simulink model "TCM8AMPM_4QAM"  (Simulink 10.2)
settings: Solver=VariableStepDiscrete  StartTime=0.0  StopTime=1e5  RelTol=1e-3  EnableMultiTasking=on
model workspace (MAT data in the model file):
  A = 1
  BER_exit = 0.0020497950205
  BER_th = 0.001
  K = 4
  M = 8
  N = 50
  P_TCM = 10
  P_UNCODED = 2
  T = 1
  ber_TCM = [0.36658979244 0.35791637421 0.332748420736 0.291837962499 0.223052241051 0.119372305224 0.0331896119523 0.00376015241151 0.000300812192921 0.000100270730974]
  ber_UNCODED = [0.163933606639 0.133536646335 0.104839516048 0.0776922307769 0.0546445355464 0.035696430357 0.0220477952205 0.012398760124 0.00599940005999 0.0020497950205]
  ber_tcm_bit_coded = [0.423343026171 0.416825428657 0.395217086133 0.359671112002 0.293291888098 0.173568635315 0.0536448410709 0.00681840970621 0 0]
  ber_tcm_bit_uncoded = [0.104791258055 0.0724912090885 0.0548450565667 0.0454348766768 0.0279695521331 0.0128376571276 0.00521455730581 0.00212593642438 0.000601624385842 0.000200541461947]
  coded_bit = 2
  coded_bit_conv = [2 3]
  codegen = [1  0  0; 0  133  171]
  codegen_2 = [133 171]
  constlen = [1 7]
  constlen_2 = 7
  generator_c1 = 133
  generator_c2 = 171
  h = 22
  hh = 0
  hws = Simulink.ModelWorkspace
  i = 11
  k = 2
  label_coded = 'TCM8AMPM'
  label_uncoded = '4QAM'
  list : struct (value not decoded)
  m = 3
  mapping_tcm = [-1+3i 3-1i 3+3i -1-1i -3+1i 1-3i 1+1i -3-3i]
  mdl_name = 'TCM8AMPM_4QAM'
  mm = 0
  n = 10000
  num_states = 64
  register_length = 7
  seed = 208004
  snr = 10
  snr_start = 0
  snr_step = 1
  snr_vec = [0 1 2 3 4 5 6 7 8 9 10]
  ss = 0.49
  startTime = [2021 6 12 8 24 9.036]
  stepTime = [2021 6 12 8 25 8.076]
  step_dur = 0.49
  tb = 28
  tout = [9001 9002 9003 9004 9005 9006 9007 9008 9009 9010 9011 9012 ... (1000 elements, 1000x1)]
  trellis.numInputSymbols = 4
  trellis.numOutputSymbols = 8
  trellis.numStates = 64
  trellis.nextStates = [0  32  0  32; 0  32  0  32; 1  33  1  33; 1  33  1  33; 2  34  2  34; 2  34  2  34; 3  35  3  35; 3  35  3  35; 4  36  4  36; 4  36  4  36; 5  37  5  37; 5  37  5  37; 6  38  6  38; 6  38  6  38; 7  39  7  39; 7  39  7  39; 8  40  8  40; 8  40  8  40; 9  41  9  41; 9  41  9  41; 10  42  10  42; 10  42  10  42; 11  43  11  43; 11  43  11  43; 12  44  12  44; 12  44  12  44; 13  45  13  45; 13  45  13  45; 14  46  14  46; 14  46  14  46; 15  47  15  47; 15  47  15  47; 16  48  16  48; 16  48  16  48; 17  49  17  49; 17  49  17  49; 18  50  18  50; 18  50  18  50; 19  51  19  51; 19  51  19  51; 20  52  20  52; 20  52  20  52; 21  53  21  53; 21  53  21  53; 22  54  22  54; 22  54  22  54; 23  55  23  55; 23  55  23  55; 24  56  24  56; 24  56  24  56; 25  57  25  57; 25  57  25  57; 26  58  26  58; 26  58  26  58; 27  59  27  59; 27  59  27  59; 28  60  28  60; 28  60  28  60; 29  61  29  61; 29  61  29  61; 30  62  30  62; 30  62  30  62; 31  63  31  63; 31  63  31  63]
  trellis.outputs = [0  3  4  7; 3  0  7  4; 2  1  6  5; 1  2  5  6; 0  3  4  7; 3  0  7  4; 2  1  6  5; 1  2  5  6; 3  0  7  4; 0  3  4  7; 1  2  5  6; 2  1  6  5; 3  0  7  4; 0  3  4  7; 1  2  5  6; 2  1  6  5; 3  0  7  4; 0  3  4  7; 1  2  5  6; 2  1  6  5; 3  0  7  4; 0  3  4  7; 1  2  5  6; 2  1  6  5; 0  3  4  7; 3  0  7  4; 2  1  6  5; 1  2  5  6; 0  3  4  7; 3  0  7  4; 2  1  6  5; 1  2  5  6; 1  2  5  6; 2  1  6  5; 3  0  7  4; 0  3  4  7; 1  2  5  6; 2  1  6  5; 3  0  7  4; 0  3  4  7; 2  1  6  5; 1  2  5  6; 0  3  4  7; 3  0  7  4; 2  1  6  5; 1  2  5  6; 0  3  4  7; 3  0  7  4; 2  1  6  5; 1  2  5  6; 0  3  4  7; 3  0  7  4; 2  1  6  5; 1  2  5  6; 0  3  4  7; 3  0  7  4; 1  2  5  6; 2  1  6  5; 3  0  7  4; 0  3  4  7; 1  2  5  6; 2  1  6  5; 3  0  7  4; 0  3  4  7]
  trellis_2.numInputSymbols = 2
  trellis_2.numOutputSymbols = 4
  trellis_2.numStates = 64
  trellis_2.nextStates = [0  32; 0  32; 1  33; 1  33; 2  34; 2  34; 3  35; 3  35; 4  36; 4  36; 5  37; 5  37; 6  38; 6  38; 7  39; 7  39; 8  40; 8  40; 9  41; 9  41; 10  42; 10  42; 11  43; 11  43; 12  44; 12  44; 13  45; 13  45; 14  46; 14  46; 15  47; 15  47; 16  48; 16  48; 17  49; 17  49; 18  50; 18  50; 19  51; 19  51; 20  52; 20  52; 21  53; 21  53; 22  54; 22  54; 23  55; 23  55; 24  56; 24  56; 25  57; 25  57; 26  58; 26  58; 27  59; 27  59; 28  60; 28  60; 29  61; 29  61; 30  62; 30  62; 31  63; 31  63]
  trellis_2.outputs = [0  3; 3  0; 2  1; 1  2; 0  3; 3  0; 2  1; 1  2; 3  0; 0  3; 1  2; 2  1; 3  0; 0  3; 1  2; 2  1; 3  0; 0  3; 1  2; 2  1; 3  0; 0  3; 1  2; 2  1; 0  3; 3  0; 2  1; 1  2; 0  3; 3  0; 2  1; 1  2; 1  2; 2  1; 3  0; 0  3; 1  2; 2  1; 3  0; 0  3; 2  1; 1  2; 0  3; 3  0; 2  1; 1  2; 0  3; 3  0; 2  1; 1  2; 0  3; 3  0; 2  1; 1  2; 0  3; 3  0; 1  2; 2  1; 3  0; 0  3; 1  2; 2  1; 3  0; 0  3]
  uncoded_bit = 1
undefined symbols (not defined in the file): Mnum
libraries: commsink2 x4, commutil2 x4, dspindex x4, commdigbbndam3 x3, commchan3 x2, commcnvcod2 x2, commdigbbndtcm2 x1, commrandsrc2 x1
settings Model: Creator=Diego  LastModifiedBy=diego
settings DataIOCC: LimitDataPoints=on
settings OptimizationCC: ExpressionDepthLimit=2147483647
settings DebuggingCC: SolverPrmCheckMsg=warning  StateNameClashWarn=warning
settings GRTTargetCC: CombineOutputUpdateFcns=on  GRTInterface=off

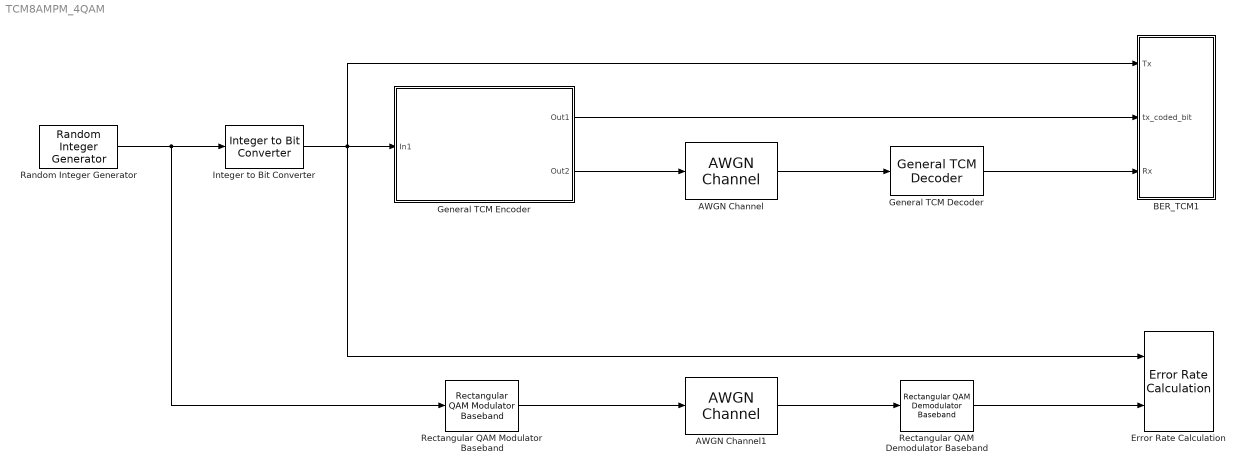
== system TCM8AMPM_4QAM ==
  AWGN Channel : commchan3/AWGN Channel  InputProcessing=Columns as channels (frame based)  seed=seed  noiseMode="Signal to noise ratio  (Es/No)"  EbNodB=Eb_No  EsNodB=snr  SNRdB=snr  bitsPerSym=k  Ps=P_TCM  Tsym=T  variance=1
  AWGN Channel1 : commchan3/AWGN Channel  InputProcessing=Columns as channels (frame based)  seed=seed  noiseMode="Signal to noise ratio  (Es/No)"  EbNodB=Eb_No  EsNodB=snr  SNRdB=snr  bitsPerSym=k  Ps=P_UNCODED  Tsym=T  variance=1
  BER_TCM1 : Subsystem
  Error Rate Calculation : commsink2/Error Rate Calculation  N=0  st_delay=0  cp_mode=Entire frame  subframe=[]  PMode=Workspace  WsName=ErrorVec_UNCODED  RsMode2=off  stop=off  numErr=100  maxBits=1e7
  General TCM Decoder : commdigbbndtcm2/General TCM Decoder  trellis=trellis  constpts=mapping_tcm  tbdepth=tb  opmode=Continuous  reset=off  outDtype=double
      settings: SourceProductBaseCode=CM
  General TCM Encoder : Subsystem  AncestorBlock=commdigbbndtcm2/General TCM Encoder  mask(General TCM Encoder){trellis=trellis, opMode=Continuous, constpts=mapping_tcm, outDtype=double}
      mask prompts: trellis "Trellis structure:"; opMode "Operation mode:"; constpts "Signal constellation:"; outDtype "Output data type"
      mask help:
      | Convolutionally encode binary data and perform signal mapping using the Signal constellation parameter, which expects complex constellation points in the set-partitioned order.
      |
      | The Trellis structure parameter must be a valid MATLAB trellis structure. To check if a structure is a valid trellis structure, use the istrellis function in MATLAB.
      mask init:
      | [constpts, Mnum, err, inPortLbl, rstPortLbl] = commblkgentcmenc(gcb, 'init', trellis, constpts);
      | if ~isempty(err.msg)
      | 	error(err.mmi,err.msg);
      | end
      mask Help: helpview(commbhelp)
      mask TypeOptions opMode: Continuous | Truncated (reset every frame) | Terminate trellis by appending bits | Reset on nonzero input via port
      mask TypeOptions outDtype: double | single
      mask Callback outDtype: commblkgentcmenc(gcb, 'cbDtype');
      mask Display:
      | disp('General\nTCM');
      | text(inPortLbl.x, inPortLbl.y, inPortLbl.str);
      | text(rstPortLbl.x, rstPortLbl.y, rstPortLbl.str);
  Integer to Bit Converter : commutil2/Integer to Bit Converter  nbits=2  signedInputValues=Unsigned  bitOrder=MSB first  outDtype=Inherit via internal rule
  Random Integer Generator : commrandsrc2/Random Integer Generator  mul=4  seed=10  Ts=1  frameBased=off  sampPerFrame=1000  orient=off  outDataType=double
      settings: SourceProductBaseCode=CM
  Rectangular QAM Demodulator Baseband : commdigbbndam3/Rectangular QAM Demodulator Baseband  M=4  OutType=Bit  DecType=Hard decision  VarSource=Dialog  Variance=1  Dec=Gray  Mapping=[0:15]  PowType=Min. distance between symbols  MinDist=2  AvgPow=1  PeakPow=1  Ph=0  outDtype1=Inherit via internal rule  outDtype2=Inherit via internal rule  derotateFactorWordLen=16  derotateFactorDataTypeStr=Inherit: Same word length as input  derotateFactorLastDataTypeStr=Inherit: Same word length as input  denormFactorWordLen=16  denormFactorDataTypeStr=Inherit: Same word length as input  denormFactorLastDataTypeStr=Inherit: Same word length as input  prodOutWordLen=32  prodOutOverflowMode=Wrap  prodOutRoundingMode=Floor  prodOutOvFlMode=off  prodOutOvFlModeLastStrValue=off  sumWordLen=32
  Rectangular QAM Modulator Baseband : commdigbbndam3/Rectangular QAM Modulator Baseband  M=4  InType=Integer  Enc=Gray  Mapping=[0:15]  PowType=Min. distance between symbols  MinDist=2  AvgPow=1  PeakPow=1  Ph=0  outDtype=double  outWordLen=16  outUDDataType=sfix(16)  outFracLenMode=Best precision  outFracLen=15  outDataTypeStr=double  outLastDataTypeStr=double
  wires:
  Integer to Bit Converter/1 -> Error Rate Calculation/1, General TCM Encoder/1(In1), BER_TCM1/1(Tx)
  Random Integer Generator/1 -> Rectangular QAM Modulator Baseband/1, Integer to Bit Converter/1
  AWGN Channel/1 -> General TCM Decoder/1
  General TCM Decoder/1 -> BER_TCM1/3(Rx)
  Rectangular QAM Modulator Baseband/1 -> AWGN Channel1/1
  AWGN Channel1/1 -> Rectangular QAM Demodulator Baseband/1
  Rectangular QAM Demodulator Baseband/1 -> Error Rate Calculation/2
  General TCM Encoder/2(Out2) -> AWGN Channel/1
  General TCM Encoder/1(Out1) -> BER_TCM1/2(tx_coded_bit)

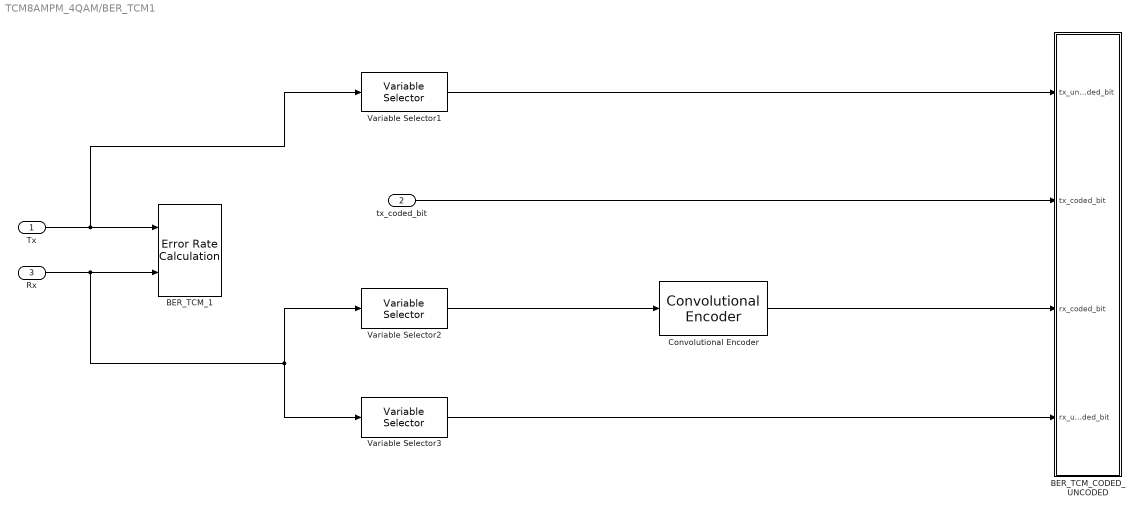
== system TCM8AMPM_4QAM/BER_TCM1 ==
  Tx : Inport
  tx_coded_bit : Inport  Port=2
  Rx : Inport  Port=3
  BER_TCM_1 : commsink2/Error Rate Calculation  N=tb*k  st_delay=0  cp_mode=Entire frame  subframe=[]  PMode=Workspace  WsName=ErrorVec_TCM_1  RsMode2=off  stop=off  numErr=100  maxBits=1e6
  BER_TCM_CODED_UNCODED : Subsystem
  Convolutional Encoder : commcnvcod2/Convolutional Encoder  trellis=trellis_2  opMode=Continuous  DelayedResetAction=off  hasIniStPort=off  hasFinStPort=off  usePuncVector=off  punctureVector=[1; 1; 0; 1; 0; 1]  reset=Unused parameter value
      settings: SourceProductBaseCode=CM
  Variable Selector1 : dspindex/Variable Selector  NumInputs=1  rowsOrCols=Rows  IdxMode=Fixed  Elements=uncoded_bit  ZerOneIdxMode=One-based  errmode=Clip Index  FillMode=on  FillValues=0
  Variable Selector2 : dspindex/Variable Selector  NumInputs=1  rowsOrCols=Rows  IdxMode=Fixed  Elements=coded_bit  ZerOneIdxMode=One-based  errmode=Clip Index  FillMode=on  FillValues=0
  Variable Selector3 : dspindex/Variable Selector  NumInputs=1  rowsOrCols=Rows  IdxMode=Fixed  Elements=uncoded_bit  ZerOneIdxMode=One-based  errmode=Clip Index  FillMode=on  FillValues=0
  wires:
  Tx/1 -> BER_TCM_1/1, Variable Selector1/1
  Rx/1 -> BER_TCM_1/2, Variable Selector2/1, Variable Selector3/1
  Variable Selector1/1 -> BER_TCM_CODED_UNCODED/1(tx_uncoded_bit)
  Variable Selector2/1 -> Convolutional Encoder/1
  Variable Selector3/1 -> BER_TCM_CODED_UNCODED/4(rx_uncoded_bit)
  tx_coded_bit/1 -> BER_TCM_CODED_UNCODED/2(tx_coded_bit)
  Convolutional Encoder/1 -> BER_TCM_CODED_UNCODED/3(rx_coded_bit)

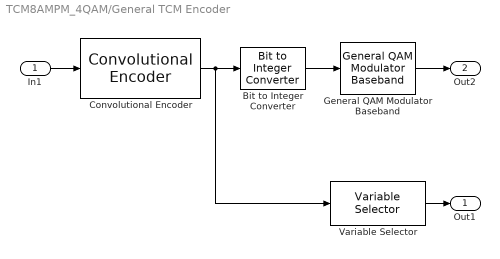
== system TCM8AMPM_4QAM/General TCM Encoder ==
  In1 : Inport
  Bit to Integer Converter : commutil2/Bit to Integer Converter  nbits=log2(Mnum)  bitOrder=MSB first  signedOutputValues=Unsigned  outDtype=uint32  outDtypeSigned=Inherit via internal rule
  Convolutional Encoder : commcnvcod2/Convolutional Encoder  trellis=trellis  opMode=Continuous  DelayedResetAction=off  hasIniStPort=off  hasFinStPort=off  usePuncVector=off  punctureVector=[1; 1; 0; 1; 0; 1]  reset=Unused parameter value
      settings: SourceProductBaseCode=CM
  General QAM Modulator Baseband : commdigbbndam3/General QAM Modulator Baseband  SigCon=constpts  outDtype=double  outWordLen=16  outUDDataType=sfix(16)  outFracLenMode=Best precision  outFracLen=15  outDataTypeStr=double  outLastDataTypeStr=double
      settings: SourceProductBaseCode=CM
  Variable Selector : dspindex/Variable Selector  NumInputs=1  rowsOrCols=Rows  IdxMode=Fixed  Elements=coded_bit_conv  ZerOneIdxMode=One-based  errmode=Clip Index  FillMode=on  FillValues=0
  Out1 : Outport
  Out2 : Outport  Port=2
  wires:
  Bit to Integer Converter/1 -> General QAM Modulator Baseband/1
  In1/1 -> Convolutional Encoder/1
  Convolutional Encoder/1 -> Bit to Integer Converter/1, Variable Selector/1
  General QAM Modulator Baseband/1 -> Out2/1
  Variable Selector/1 -> Out1/1

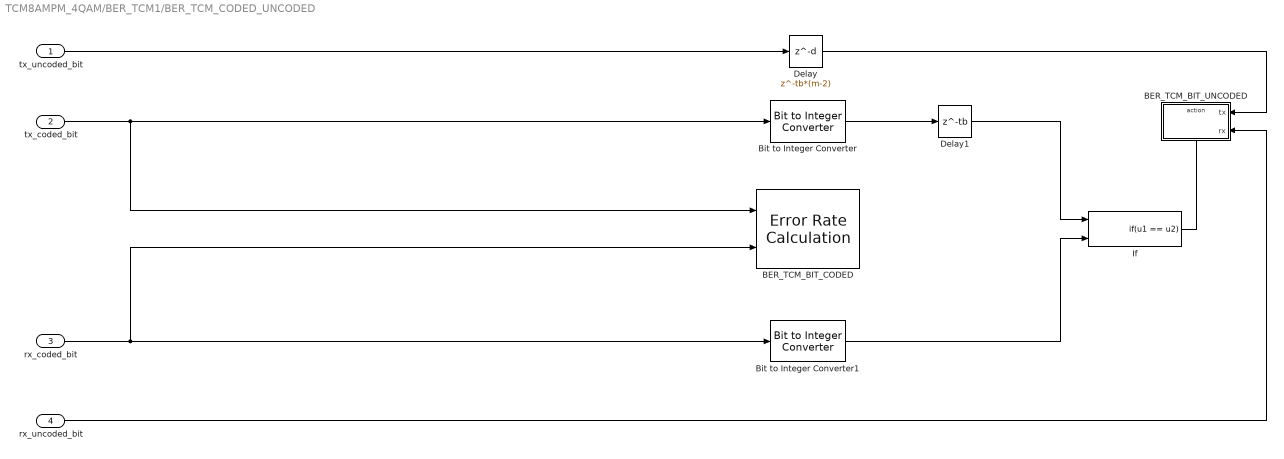
== system TCM8AMPM_4QAM/BER_TCM1/BER_TCM_CODED_UNCODED ==
  tx_uncoded_bit : Inport
  tx_coded_bit : Inport  Port=2
  rx_coded_bit : Inport  Port=3
  rx_uncoded_bit : Inport  Port=4
  BER_TCM_BIT_CODED : commsink2/Error Rate Calculation  N=tb*2  st_delay=0  cp_mode=Entire frame  subframe=[]  PMode=Workspace  WsName=ErrorVec_TCM_COD_1  RsMode2=off  stop=off  numErr=100  maxBits=1e6
  BER_TCM_BIT_UNCODED : Subsystem  TreatAsAtomicUnit=on
  Bit to Integer Converter : commutil2/Bit to Integer Converter  nbits=2  bitOrder=MSB first  signedOutputValues=Unsigned  outDtype=Inherit via internal rule  outDtypeSigned=Inherit via internal rule
  Bit to Integer Converter1 : commutil2/Bit to Integer Converter  nbits=2  bitOrder=MSB first  signedOutputValues=Unsigned  outDtype=Inherit via internal rule  outDtypeSigned=Inherit via internal rule
  Delay : Delay  DelayLength=tb*(m-2)  InputProcessing=Columns as channels (frame based)
  Delay1 : Delay  DelayLength=tb  InputProcessing=Columns as channels (frame based)
  If : If  NumInputs=2  IfExpression=u1 == u2  ShowElse=off
  wires:
  tx_uncoded_bit/1 -> Delay/1
  tx_coded_bit/1 -> BER_TCM_BIT_CODED/1, Bit to Integer Converter/1
  rx_coded_bit/1 -> BER_TCM_BIT_CODED/2, Bit to Integer Converter1/1
  Delay/1 -> BER_TCM_BIT_UNCODED/1(tx)
  rx_uncoded_bit/1 -> BER_TCM_BIT_UNCODED/2(rx)
  If/1 -> BER_TCM_BIT_UNCODED/Action
  Bit to Integer Converter/1 -> Delay1/1
  Bit to Integer Converter1/1 -> If/2
  Delay1/1 -> If/1

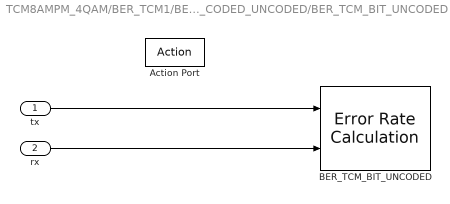
== system TCM8AMPM_4QAM/BER_TCM1/BER_TCM_CODED_UNCODED/BER_TCM_BIT_UNCODED ==
  tx : Inport
  rx : Inport  Port=2
  Action Port : ActionPort  ActionPortLabel=if(u1 == u2)
  BER_TCM_BIT_UNCODED : commsink2/Error Rate Calculation  N=0  st_delay=tb*(m-2)  cp_mode=Entire frame  subframe=[]  PMode=Workspace  WsName=ErrorVec_TCM_bit_uncoded  RsMode2=off  stop=off  numErr=100  maxBits=1e6
  wires:
  tx/1 -> BER_TCM_BIT_UNCODED/1
  rx/1 -> BER_TCM_BIT_UNCODED/2
